simulink model "sending_app1"  (R2022b)
settings: Solver=FixedStepAuto  StartTime=0.0  StopTime=inf  FixedStep=0.0125  RelTol=1e-3
libraries: androiduilib x8, androidaudiovideolib x3, androidcommunicationlib x3, androidsensorlib x2, fuzblock x1
settings Model: Creator=Akshat  LastModifiedBy=Akshat
settings OptimizationCC: EnhancedBackFolding=on  PassReuseOutputArgsAs=Individual arguments  ZeroExternalMemoryAtStartup=off  ZeroInternalMemoryAtStartup=off  MaxStackSize=64  OptimizeBlockOrder=speed  DifferentSizesBufferReuse=on  OptimizationCustomize=off  EfficientTunableParamExpr=on
settings DebuggingCC: ParameterTunabilityLossMsg=error
settings HardwareCC: ProdBitPerPointer=32  ProdBitPerSizeT=32  ProdBitPerPtrDiffT=32  ProdLargestAtomicInteger=Long  ProdLargestAtomicFloat=Double  ProdWordSize=32  ProdHWDeviceType=ARM Compatible->ARM Cortex  UseEmbeddedCoderFeatures=off
settings SFSimCC: MATLABDynamicMemAlloc=off
settings RTWCC: Description=Embedded Coder  SystemTargetFile=ert.tlc  HardwareBoard=Android Device  TLCOptions="-aInlineSetEventsForThisBaseRateFcn=TLC_FALSE -aSuppressMultiTaskScheduler=TLC_FALSE  -aRateBasedStepFcn=0"  TemplateMakefile=ert_default_tmf  RTWVerbose=off  Toolchain=Android SDK/NDK Tools
settings CodeAppCC: ForceParamTrailComments=on  IgnoreCustomStorageClasses=off  OperatorAnnotations=on  SimulinkDataObjDesc=on  SFDataObjDesc=on  InsertBlockDesc=on
settings ERTTargetCC: SupportNonInlinedSFcns=on

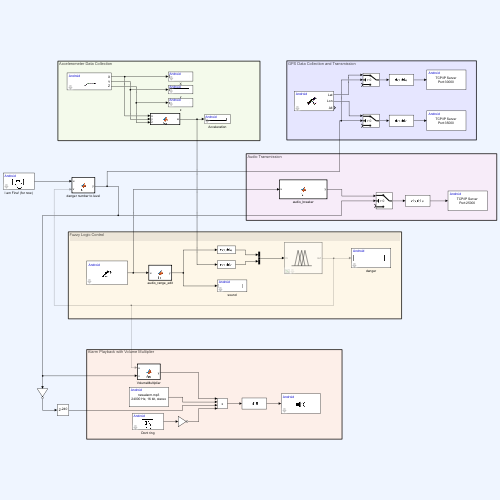
[thumbnail: Simulink's stored preview of the top-level diagram]
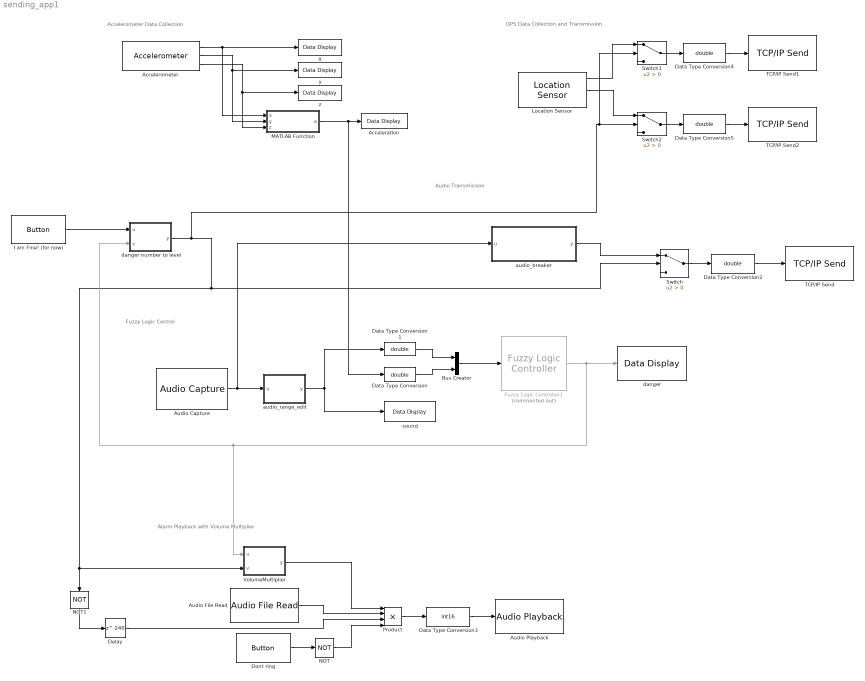
== system sending_app1 ==
  note: Audio Transmission
  note: Fuzzy Logic Control
  note: Alarm Playback with Volume Multiplier
  note: GPS Data Collection and Transmission
  note: Accelerometer Data Collection
  Acceleration : androiduilib/Data Display  DataDisplayId=sending_app1/Acceleration  Format=Float  Precision=6  SimulateUsing=Code generation  blockPlatform=Android
  Accelerometer : androidsensorlib/Accelerometer  OutputVector=off  SampleTime=0.1  BlockPlatform=Android
  Audio Capture : androidaudiovideolib/Audio Capture  SampleFreq=24000  FrameSize=300  SampleTime=0.0125  SimulateUsing=Code generation  DeviceStr=0  QueueDuration=0  BlockPlatform=Android  AudioSamplingFreq=44100
  Audio File Read : androidaudiovideolib/Audio File Read  FileName=D:\Courses\ES245_ControlSystems\newalarm.mp3  FrameSize=300
  Audio Playback : androidaudiovideolib/Audio Playback  SampleFreq=24000  AudioSamplingFreq=24000  SampleTime=0.1  DeviceStr=0  QueueDuration=0  BlockPlatform=Android
  Bus Creator : BusCreator  Inputs=2
  Data Type Conversion{,1..2,4..5} (5 alike) : DataTypeConversion  OutDataTypeStr=double  SaturateOnIntegerOverflow=off  RndMeth=Floor
  Data Type Conversion3 : DataTypeConversion  OutDataTypeStr=int16  SaturateOnIntegerOverflow=off  RndMeth=Floor
  Delay : Delay  DelayLength=240
  Dont ring : androiduilib/Button  ButtonState=Not pressed  ButtonId=sending_app1/Dont_ring  State=off  SampleTime=0.0125  BlockPlatform=Android
  Fuzzy Logic Controller1 : fuzblock/Fuzzy Logic  Controller  Commented=on  FIS=fuzzy_verylow  OutputSampleNumber=101  DataType=double  FuzzifiedInputs=off  RuleFiringStrengths=off  RuleOutputs=off  AggregatedOutputs=off  SimulateUsing=Interpreted execution  OutOfRangeInputValueMessage=warning  NoRuleFiredMessage=warning  EmptyOutputFuzzySetMessage=warning
  I am Fine! (for now) : androiduilib/Button  ButtonState=Not pressed  ButtonId=sending_app1/I_am_Fine!_(for_now)  State=off  SampleTime=0.1  BlockPlatform=Android
  Location Sensor : androidsensorlib/Location Sensor  OutputVector=off  SampleTime=0.0125  BlockPlatform=Android
  MATLAB Function : MATLAB Function  TreatAsAtomicUnit=on
  NOT : Logic  Operator=NOT  IconShape=distinctive  AllPortsSameDT=off  OutDataTypeStr=boolean
  NOT1 : Logic  Operator=NOT  IconShape=distinctive  AllPortsSameDT=off  OutDataTypeStr=boolean
  Product : Product  Inputs=4
  Switch : Switch  Criteria=u2 > Threshold  SaturateOnIntegerOverflow=off  InputSameDT=off
  Switch1 : Switch  Criteria=u2 > Threshold  OutDataTypeStr=double  SaturateOnIntegerOverflow=off  InputSameDT=off
  Switch2 : Switch  Criteria=u2 > Threshold  OutDataTypeStr=double  SaturateOnIntegerOverflow=off  InputSameDT=off
  TCP/IP Send : androidcommunicationlib/TCP//IP Send  TCPSendId=sending_app1/TCP//IP_Send  Mode_=Server  LocalServerPort_=25000  RemoteAddr_=10.7.21.239  RemoteServerPort_=25000  ClientPortBindingSelection_=off  ClientPortToBind_=35000  BlockingMode_=off  BlockTimeout_=0.1
  TCP/IP Send1 : androidcommunicationlib/TCP//IP Send  TCPSendId=sending_app1/TCP//IP_Send1  Mode_=Server  LocalServerPort_=30000  RemoteAddr_=127.0.0.1  RemoteServerPort_=25000  ClientPortBindingSelection_=off  ClientPortToBind_=35000  BlockingMode_=off  BlockTimeout_=0.1
  TCP/IP Send2 : androidcommunicationlib/TCP//IP Send  TCPSendId=sending_app1/TCP//IP_Send2  Mode_=Server  LocalServerPort_=35000  RemoteAddr_=127.0.0.1  RemoteServerPort_=25000  ClientPortBindingSelection_=off  ClientPortToBind_=35000  BlockingMode_=off  BlockTimeout_=0.1
  VolumeMultiplier : MATLAB Function  TreatAsAtomicUnit=on
  X : androiduilib/Data Display  DataDisplayId=sending_app1/X  Format=Float  Precision=6  SimulateUsing=Code generation  blockPlatform=Android
  audio_breaker : MATLAB Function  TreatAsAtomicUnit=on
  audio_range_edit : MATLAB Function  TreatAsAtomicUnit=on
  danger : androiduilib/Data Display  DataDisplayId=sending_app1/danger  Format=Float  Precision=6  SimulateUsing=Code generation  blockPlatform=Android
  "danger number to level " : MATLAB Function  TreatAsAtomicUnit=on
  sound : androiduilib/Data Display  DataDisplayId=sending_app1/sound  Format=Float  Precision=6  SimulateUsing=Code generation  blockPlatform=Android
  y : androiduilib/Data Display  DataDisplayId=sending_app1/y  Format=Float  Precision=6  SimulateUsing=Code generation  blockPlatform=Android
  z : androiduilib/Data Display  DataDisplayId=sending_app1/z  Format=Float  Precision=6  SimulateUsing=Code generation  blockPlatform=Android
  wires:
  Accelerometer/1 -> MATLAB Function/1(x), X/1
  Accelerometer/2 -> MATLAB Function/2(y), y/1
  Accelerometer/3 -> MATLAB Function/3(z), z/1
  MATLAB Function/1(a) -> Data Type Conversion/1, Acceleration/1
  Bus Creator/1 -> Fuzzy Logic Controller1/1
  Audio Capture/1 -> audio_breaker/1(u), audio_range_edit/1(u)
  audio_range_edit/1(y) -> Data Type Conversion1/1, sound/1
  Data Type Conversion/1 -> Bus Creator/2
  Data Type Conversion1/1 -> Bus Creator/1
  Switch/1 -> Data Type Conversion2/1
  "danger number to level "/1(y) -> NOT1/1, VolumeMultiplier/2(v), Switch/2, Switch1/2, Switch2/2
  audio_breaker/1(y) -> Switch/1
  Data Type Conversion2/1 -> TCP/IP Send/1
  I am Fine! (for now)/1 -> "danger number to level "/1(u)
  VolumeMultiplier/1(y) -> Product/1
  Product/1 -> Data Type Conversion3/1
  Audio File Read/1 -> Product/2
  Data Type Conversion3/1 -> Audio Playback/1
  Dont ring/1 -> NOT/1
  NOT/1 -> Product/4
  Switch1/1 -> Data Type Conversion4/1
  Location Sensor/1 -> Switch1/1
  Data Type Conversion4/1 -> TCP/IP Send1/1
  Switch2/1 -> Data Type Conversion5/1
  Data Type Conversion5/1 -> TCP/IP Send2/1
  Location Sensor/2 -> Switch2/1
  NOT1/1 -> Delay/1
  Fuzzy Logic Controller1/1 -> VolumeMultiplier/1(u), "danger number to level "/2(v), danger/1
  Delay/1 -> Product/3

== matlab function sending_app1/MATLAB Function ==
  data: x input; a output; y input; z input
function a = fcn(x,y,z)
x = x/60;
y = y/80;
z = z/80;

ai = (x^2)+(y^2)+(z^2);
b = ai^0.5;
a = b;

== matlab function sending_app1/audio_breaker ==
  data: u input; y output
function y = fcn(u)
y = u(:,1);

== matlab function sending_app1/danger number to level  ==
  data: u input; y output; v input
function y = fcn(u,v)
persistent flag;

    if isempty(flag)
        flag = 0;
    end

    if u == 1
        flag = 0;
        y = 0;
    elseif v > 0.45
        flag = 1;
        y = 1;
    else
        y = flag;
    end
end

== matlab function sending_app1/VolumeMultiplier ==
  data: u input; y output; v input
function y = fcn(u, v)
    if v ==1
               y = 1;
    elseif u < 0.25
        y = 0;
    elseif u >= 0.20 && u < 0.35
        y = 0.2;
    else
        y = 1;
    end

== matlab function sending_app1/audio_range_edit ==
  data: u input; y output
function y = fcn(u)
ui = abs(u);
yi = mean(ui,2);
y = mean(yi)/20000;
